simulink model "testmodel_3"  (R2018b)
settings: Solver=VariableStepAuto  StartTime=0.0  StopTime=20  RelTol=1e-3
values from neighbouring files (symbols this model uses):
  Gain_brain = 20    [Model_versie_1.m]
  k_1 = 1/K_g    (= 1.26582278481)    [Model_versie_1.m]    (also in Model_versie_5_clean.m)
  mu = 5    [Model_versie_1.m]    (also in Model_versie_5_clean.m = B_g/(2*sqrt(K_g*J_g)))
  Time_delay = 0.00    (= 0)    [Model_versie_1.m]    (also in Model_versie_5_clean.m = 0.01)
  Tp = 0.037    [Model_versie_1.m]
  wn = 120    [Model_versie_1.m]    (also in Model_versie_5_clean.m = sqrt(K_g/J_g))
settings Model: Creator=janwi  LastModifiedBy=janwi
settings SimscapeCC: SimscapeLogType=all

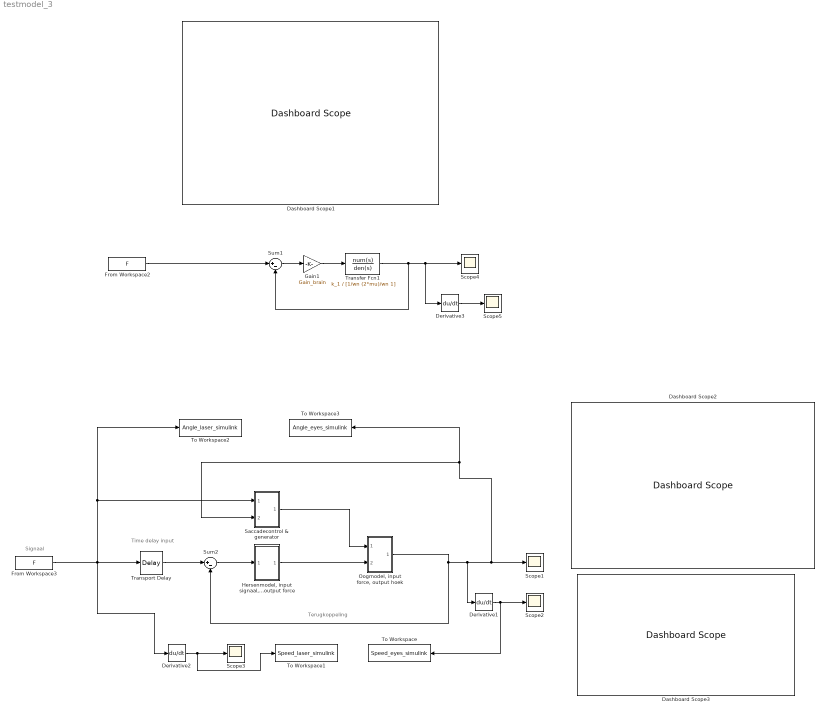
== system testmodel_3 ==
  note: Terugkoppeling
  note: Signaal
  note: Time delay input
  Dashboard Scope1 : DashboardScope  WebBlockId=93
  Dashboard Scope2 : DashboardScope  WebBlockId=117
  Dashboard Scope3 : DashboardScope  WebBlockId=132
  Derivative1 : Derivative  CoefficientInTFapproximation=1
  Derivative2 : Derivative  CoefficientInTFapproximation=1
  Derivative3 : Derivative  CoefficientInTFapproximation=1
  From Workspace2 : FromWorkspace  VariableName=F  SampleTime=0
  From Workspace3 : FromWorkspace  VariableName=F  SampleTime=0
  Gain1 : Gain  Gain=Gain_brain
  "Hersenmodel, input signaal, output force" : Subsystem
  "Oogmodel, input force, output hoek" : Subsystem
  Saccadecontrol & generator : Subsystem
  Scope{1..5} (5 alike) : Scope
  Sum1 : Sum  Inputs=|+-
  Sum2 : Sum  Inputs=|+-
  To Workspace : ToWorkspace  VariableName=Speed_eyes_simulink  SampleTime=1e-3
      settings: Save2DSignal=2-D array (concatenate along first dimension)
  To Workspace1 : ToWorkspace  VariableName=Speed_laser_simulink  SampleTime=1e-3
      settings: Save2DSignal=2-D array (concatenate along first dimension)
  To Workspace2 : ToWorkspace  VariableName=Angle_laser_simulink  SampleTime=1e-3
      settings: Save2DSignal=2-D array (concatenate along first dimension)
  To Workspace3 : ToWorkspace  VariableName=Angle_eyes_simulink  SampleTime=1e-3
      settings: Save2DSignal=2-D array (concatenate along first dimension)
  Transfer Fcn1 : TransferFcn  Numerator=k_1  Denominator=[1/wn (2*mu)/wn 1]
  Transport Delay : TransportDelay  DelayTime=Time_delay  InitialOutput=1
  wires:
  Sum1/1 -> Gain1/1
  Gain1/1 -> Transfer Fcn1/1
  Transfer Fcn1/1 -> Derivative3/1, Scope4/1, Sum1/2
  From Workspace2/1 -> Sum1/1
  "Oogmodel, input force, output hoek"/1(Out2) -> Sum2/2, Derivative1/1, Saccadecontrol & generator/2(In3), To Workspace3/1, Scope1/1
  From Workspace3/1 -> Derivative2/1, To Workspace2/1, Saccadecontrol & generator/1(In2), Transport Delay/1
  Derivative1/1 -> Scope2/1, To Workspace/1
  Derivative2/1 -> To Workspace1/1, Scope3/1
  Derivative3/1 -> Scope5/1
  Sum2/1 -> "Hersenmodel, input signaal, output force"/1(In1)
  Transport Delay/1 -> Sum2/1
  "Hersenmodel, input signaal, output force"/1(Out1) -> "Oogmodel, input force, output hoek"/2(In1)
  Saccadecontrol & generator/1(Out1) -> "Oogmodel, input force, output hoek"/1(In2)

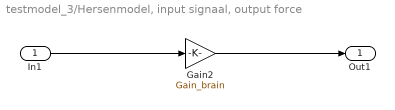
== system testmodel_3/Hersenmodel, input signaal, output force ==
  In1 : Inport
  Gain2 : Gain  Gain=Gain_brain
  Out1 : Outport
  wires:
  Gain2/1 -> Out1/1
  In1/1 -> Gain2/1

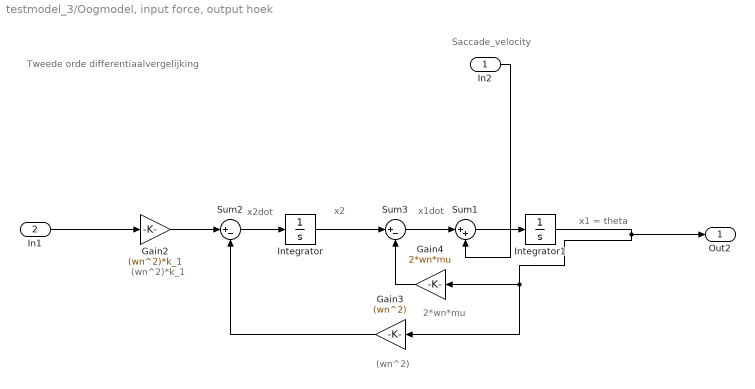
== system testmodel_3/Oogmodel, input force, output hoek ==
  note: Tweede orde differentiaalvergelijking
  note: Saccade_velocity
  note: (wn^2)*k_1
  note: 2*wn*mu
  note: (wn^2)
  note: x2dot
  note: x2
  note: x1dot
  note: x1 = theta
  In2 : Inport
  In1 : Inport  Port=2
  Gain2 : Gain  Gain=(wn^2)*k_1
  Gain3 : Gain  Gain=(wn^2)
  Gain4 : Gain  Gain=2*wn*mu
  Integrator : Integrator
  Integrator1 : Integrator
  Sum1 : Sum  Inputs=|++
  Sum2 : Sum  Inputs=|+-
  Sum3 : Sum  Inputs=|+-
  Out2 : Outport
  wires:
  Integrator1/1 -> Out2/1, Gain4/1, Gain3/1
  Gain3/1 -> Sum2/2
  Sum2/1 -> Integrator/1
  In1/1 -> Gain2/1
  Gain2/1 -> Sum2/1
  Gain4/1 -> Sum3/2
  Integrator/1 -> Sum3/1
  In2/1 -> Sum1/2
  Sum3/1 -> Sum1/1
  Sum1/1 -> Integrator1/1

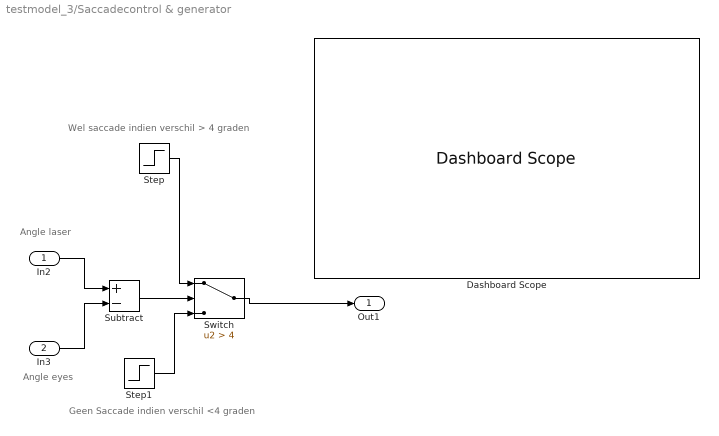
== system testmodel_3/Saccadecontrol & generator ==
  note: Wel saccade indien verschil > 4 graden
  note: Geen Saccade indien verschil <4 graden
  note: Angle laser
  note: Angle eyes
  In2 : Inport
  In3 : Inport  Port=2
  Dashboard Scope : DashboardScope  WebBlockId=184
  Step : Step  Time=Tp  After=200  SampleTime=0
  Step1 : Step  Time=Tp  After=0  SampleTime=0
  Subtract : Sum  Inputs=+-
  Switch : Switch  Criteria=u2 > Threshold  Threshold=4  ZeroCross=off
  Out1 : Outport
  wires:
  In2/1 -> Subtract/1
  In3/1 -> Subtract/2
  Subtract/1 -> Switch/2
  Step/1 -> Switch/1
  Switch/1 -> Out1/1
  Step1/1 -> Switch/3
